simulink model "NXPFRDMK64F"  (R2022a)
settings: Solver=FixedStepAuto  StartTime=0.0  StopTime=10.0  FixedStep=1e-3  RelTol=1e-3  EnableMultiTasking=on
undefined symbols (not defined in the file): D0, D1, D10, D11, D12, D13, D2, D3, D4, D5, D6, D7, D8, D9, PTA0, PTA1, PTA2, PTB23, PTB9, PTC16, PTC17, PTC2, PTC3, PTC4, PTD0, PTD1, PTD2, PTD3
libraries: frdmk64flib x16
settings Model: ExtModeTrigDuration=5  Creator=patri  LastModifiedBy=areeb
settings OptimizationCC: EnhancedBackFolding=on  PassReuseOutputArgsAs=Individual arguments  ZeroExternalMemoryAtStartup=off  ZeroInternalMemoryAtStartup=off  MaxStackSize=64  OptimizeBlockOrder=speed  DifferentSizesBufferReuse=on  OptimizationCustomize=off  EfficientTunableParamExpr=on
settings DebuggingCC: ParameterTunabilityLossMsg=error
settings HardwareCC: ProdBitPerPointer=32  ProdBitPerSizeT=32  ProdBitPerPtrDiffT=32  ProdLargestAtomicInteger=Long  ProdLargestAtomicFloat=Double  ProdWordSize=32  ProdHWDeviceType=ARM Compatible->ARM Cortex
settings SFSimCC: MATLABDynamicMemAlloc=off
settings RTWCC: SystemTargetFile=ert.tlc  HardwareBoard=NXP FRDM-K64F  TLCOptions="-aInlineSetEventsForThisBaseRateFcn=TLC_FALSE -aSuppressMultiTaskScheduler=TLC_FALSE  -aRateBasedStepFcn=0"  TemplateMakefile=ert_default_tmf  Toolchain=GNU Tools for ARM Embedded Processors
settings CodeAppCC: ForceParamTrailComments=on  IgnoreCustomStorageClasses=off  OperatorAnnotations=on  SimulinkDataObjDesc=on  SFDataObjDesc=on  InsertBlockDesc=on
settings ERTTargetCC: ExtModeTransport=4  ExtModeMexFile=sendToCommService

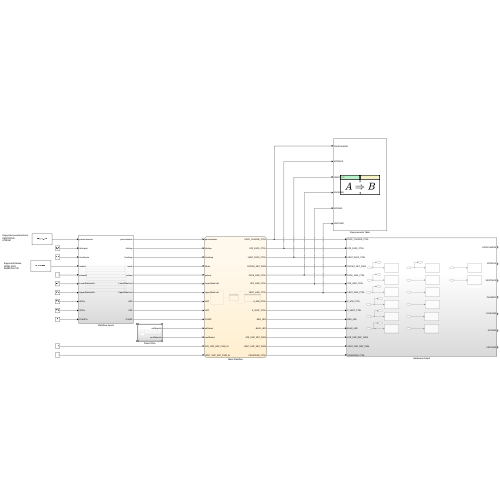
[thumbnail: Simulink's stored preview of the top-level diagram]
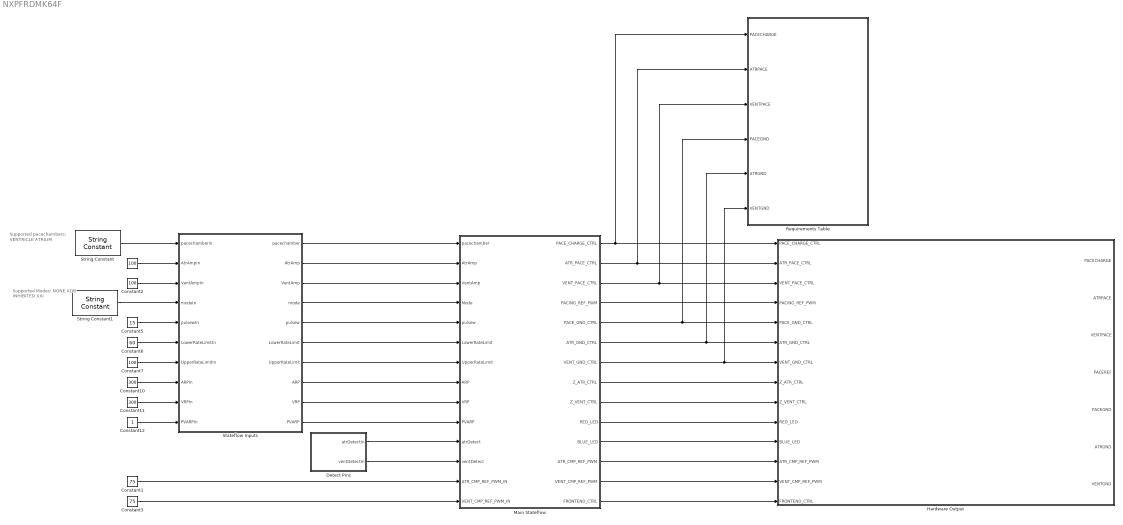
== system NXPFRDMK64F ==
  note: Supported pacechambers:
      | VENTRICLE
      | ATRIUM
  note: Supported Modes:
      | NONE XOO
      | INHIBITED XXI
  " " : Constant  Value=100
  Constant1 : Constant  Value=75
  Constant10 : Constant  Value=300
  Constant11 : Constant  Value=300
  Constant12 : Constant
  Constant2 : Constant  Value=100
  Constant3 : Constant  Value=75
  Constant5 : Constant  Value=15
  Constant6 : Constant  Value=60
  Constant7 : Constant  Value=100
  Detect Pins : Subsystem
  Hardware Output : Subsystem
  Main Stateflow : Stateflow chart  TreatAsAtomicUnit=on
  Requirements Table : Requirements Table  TreatAsAtomicUnit=on
  Stateflow Inputs : Subsystem
  String Constant : StringConstant  String="\"ATRIUM\""
  String Constant1 : StringConstant  String="\"INHIBITED\""
  wires:
  Main Stateflow/1(PACE_CHARGE_CTRL) -> Requirements Table/1(PACECHARGE), Hardware Output/1(PACE_CHARGE_CTRL)
  Main Stateflow/3(VENT_PACE_CTRL) -> Requirements Table/3(VENTPACE), Hardware Output/3(VENT_PACE_CTRL)
  Main Stateflow/4(PACING_REF_PWM) -> Hardware Output/4(PACING_REF_PWM)
  Main Stateflow/5(PACE_GND_CTRL) -> Requirements Table/4(PACEGND), Hardware Output/5(PACE_GND_CTRL)
  Main Stateflow/7(VENT_GND_CTRL) -> Requirements Table/6(VENTGND), Hardware Output/7(VENT_GND_CTRL)
  Main Stateflow/8(Z_ATR_CTRL) -> Hardware Output/8("Z_ATR_CTRL ")
  Main Stateflow/9(Z_VENT_CTRL) -> Hardware Output/9(Z_VENT_CTRL)
  Main Stateflow/11(BLUE_LED) -> Hardware Output/11(BLUE_LED)
  Main Stateflow/10(RED_LED) -> Hardware Output/10(RED_LED)
  Stateflow Inputs/1(pacechamber) -> Main Stateflow/1(pacechamber)
  Stateflow Inputs/2(AtrAmp) -> Main Stateflow/2(AtrAmp)
  Stateflow Inputs/3(VentAmp) -> Main Stateflow/3(VentAmp)
  Stateflow Inputs/4(mode) -> Main Stateflow/4(Mode)
  Stateflow Inputs/5(pulsew) -> Main Stateflow/5(pulsew)
  Stateflow Inputs/6(LowerRateLimit) -> Main Stateflow/6(LowerRateLimit)
  Stateflow Inputs/7(UpperRateLimit) -> Main Stateflow/7(UpperRateLimit)
  Stateflow Inputs/8(ARP) -> Main Stateflow/8(ARP)
  Stateflow Inputs/9(VRP) -> Main Stateflow/9(VRP)
  Stateflow Inputs/10(PVARP) -> Main Stateflow/10(PVARP)
  Detect Pins/1(atrDetectIn) -> Main Stateflow/11(atrDetect)
  Detect Pins/2(ventDetectIn) -> Main Stateflow/12(ventDetect)
  Constant12/1 -> Stateflow Inputs/10(PVARPIn)
  " "/1 -> Stateflow Inputs/2(AtrAmpIn)
  Constant2/1 -> Stateflow Inputs/3(VentAmpIn)
  String Constant1/1 -> Stateflow Inputs/4(modeIn)
  Constant5/1 -> Stateflow Inputs/5(pulsewIn)
  Constant6/1 -> Stateflow Inputs/6(LowerRateLimitIn)
  Constant7/1 -> Stateflow Inputs/7(UpperRateLimitIn)
  Constant10/1 -> Stateflow Inputs/8(ARPIn)
  Constant11/1 -> Stateflow Inputs/9(VRPIn)
  Constant1/1 -> Main Stateflow/13(ATR_CMP_REF_PWM_IN)
  Constant3/1 -> Main Stateflow/14(VENT_CMP_REF_PWM_IN)
  String Constant/1 -> Stateflow Inputs/1(pacechamberin)
  Main Stateflow/6(ATR_GND_CTRL) -> Requirements Table/5(ATRGND), Hardware Output/6(ATR_GND_CTRL)
  Main Stateflow/2(ATR_PACE_CTRL) -> Requirements Table/2(ATRPACE), Hardware Output/2(ATR_PACE_CTRL)
  Main Stateflow/12(ATR_CMP_REF_PWM) -> Hardware Output/12(ATR_CMP_REF_PWM)
  Main Stateflow/13(VENT_CMP_REF_PWM) -> Hardware Output/13(VENT_CMP_REF_PWM)
  Main Stateflow/14(FRONTEND_CTRL) -> Hardware Output/14(FRONTEND_CTRL)

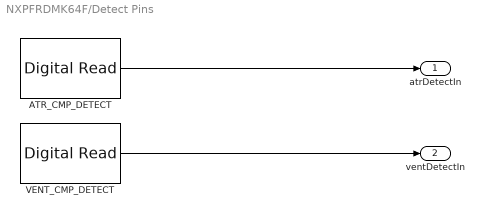
== system NXPFRDMK64F/Detect Pins ==
  ATR_CMP_DETECT : frdmk64flib/Digital Read  Whichpin=PTC16 (D0)  SampleTime=-1
  VENT_CMP_DETECT : frdmk64flib/Digital Read  Whichpin=PTC17 (D1)  SampleTime=-1
  atrDetectIn : Outport
  ventDetectIn : Outport  Port=2
  wires:
  VENT_CMP_DETECT/1 -> ventDetectIn/1
  ATR_CMP_DETECT/1 -> atrDetectIn/1

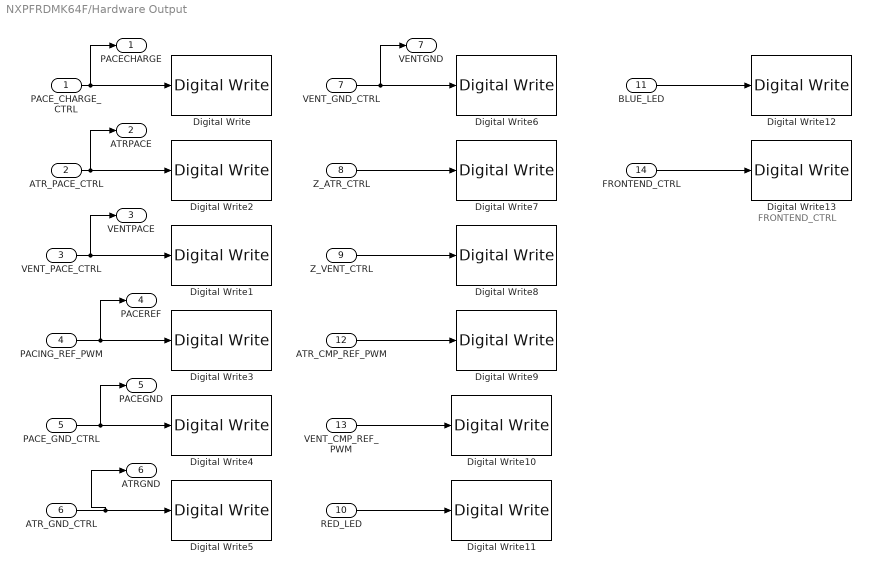
== system NXPFRDMK64F/Hardware Output ==
  note: FRONTEND_CTRL
  PACE_CHARGE_CTRL : Inport
  ATR_PACE_CTRL : Inport  Port=2
  VENT_PACE_CTRL : Inport  Port=3
  PACING_REF_PWM : Inport  Port=4
  PACE_GND_CTRL : Inport  Port=5
  ATR_GND_CTRL : Inport  Port=6
  VENT_GND_CTRL : Inport  Port=7
  "Z_ATR_CTRL " : Inport  Port=8
  Z_VENT_CTRL : Inport  Port=9
  RED_LED : Inport  Port=10
  BLUE_LED : Inport  Port=11
  ATR_CMP_REF_PWM : Inport  Port=12
  VENT_CMP_REF_PWM : Inport  Port=13
  FRONTEND_CTRL : Inport  Port=14
  Digital Write : frdmk64flib/Digital Write  Whichpin=PTB9 (D2)
  Digital Write1 : frdmk64flib/Digital Write  Whichpin=PTC4 (D9)
  Digital Write10 : frdmk64flib/Digital Write  Whichpin=PTA1 (D3)
  Digital Write11 : frdmk64flib/Digital Write  Whichpin=RED_LED
  Digital Write12 : frdmk64flib/Digital Write  Whichpin=BLUE_LED
  Digital Write13 : frdmk64flib/Digital Write  Whichpin=PTD1 (D13)
  Digital Write2 : frdmk64flib/Digital Write  Whichpin=PTA0 (D8)
  Digital Write3 : frdmk64flib/Digital Write  Whichpin=PTA2 (D5)
  Digital Write4 : frdmk64flib/Digital Write  Whichpin=PTD0 (D10)
  Digital Write5 : frdmk64flib/Digital Write  Whichpin=PTD2 (D11)
  Digital Write6 : frdmk64flib/Digital Write  Whichpin=PTD3 (D12)
  Digital Write7 : frdmk64flib/Digital Write  Whichpin=PTB23 (D4)
  Digital Write8 : frdmk64flib/Digital Write  Whichpin=PTC3 (D7)
  Digital Write9 : frdmk64flib/Digital Write  Whichpin=PTC2 (D6)
  PACECHARGE : Outport
  ATRPACE : Outport  Port=2
  VENTPACE : Outport  Port=3
  PACEREF : Outport  Port=4
  PACEGND : Outport  Port=5
  ATRGND : Outport  Port=6
  VENTGND : Outport  Port=7
  wires:
  "Z_ATR_CTRL "/1 -> Digital Write7/1
  ATR_CMP_REF_PWM/1 -> Digital Write9/1
  Z_VENT_CTRL/1 -> Digital Write8/1
  VENT_CMP_REF_PWM/1 -> Digital Write10/1
  BLUE_LED/1 -> Digital Write12/1
  PACE_CHARGE_CTRL/1 -> Digital Write/1, PACECHARGE/1
  RED_LED/1 -> Digital Write11/1
  ATR_PACE_CTRL/1 -> ATRPACE/1, Digital Write2/1
  VENT_PACE_CTRL/1 -> VENTPACE/1, Digital Write1/1
  PACING_REF_PWM/1 -> PACEREF/1, Digital Write3/1
  PACE_GND_CTRL/1 -> PACEGND/1, Digital Write4/1
  ATR_GND_CTRL/1 -> ATRGND/1, Digital Write5/1
  VENT_GND_CTRL/1 -> VENTGND/1, Digital Write6/1
  FRONTEND_CTRL/1 -> Digital Write13/1

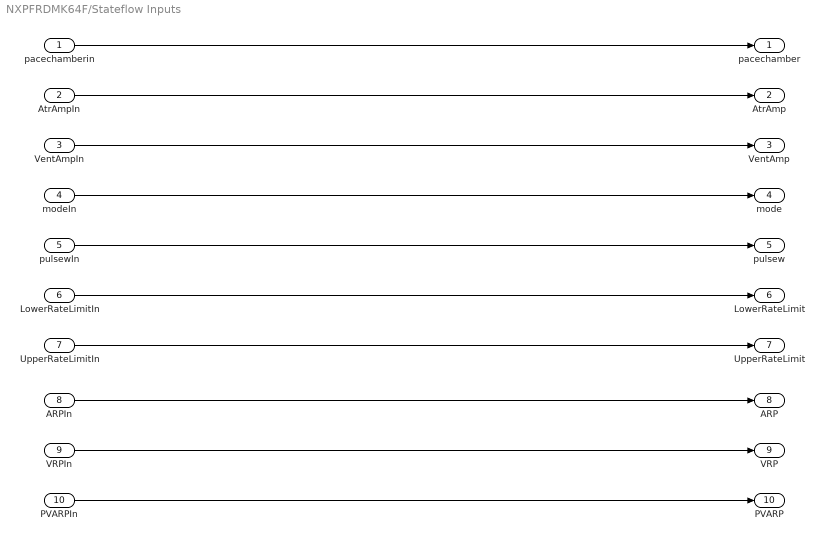
== system NXPFRDMK64F/Stateflow Inputs ==
  pacechamberin : Inport
  AtrAmpIn : Inport  Port=2
  VentAmpIn : Inport  Port=3
  modeIn : Inport  Port=4
  pulsewIn : Inport  Port=5
  LowerRateLimitIn : Inport  Port=6
  UpperRateLimitIn : Inport  Port=7
  ARPIn : Inport  Port=8
  VRPIn : Inport  Port=9
  PVARPIn : Inport  Port=10
  pacechamber : Outport
  AtrAmp : Outport  Port=2
  VentAmp : Outport  Port=3
  mode : Outport  Port=4
  pulsew : Outport  Port=5
  LowerRateLimit : Outport  Port=6
  UpperRateLimit : Outport  Port=7
  ARP : Outport  Port=8
  VRP : Outport  Port=9
  PVARP : Outport  Port=10
  wires:
  pacechamberin/1 -> pacechamber/1
  pulsewIn/1 -> pulsew/1
  modeIn/1 -> mode/1
  UpperRateLimitIn/1 -> UpperRateLimit/1
  LowerRateLimitIn/1 -> LowerRateLimit/1
  PVARPIn/1 -> PVARP/1
  AtrAmpIn/1 -> AtrAmp/1
  VentAmpIn/1 -> VentAmp/1
  ARPIn/1 -> ARP/1
  VRPIn/1 -> VRP/1

== stateflow chart NXPFRDMK64F/Requirements Table ==
  (default) -> (junction 1073742759)
  (junction 1073742759) -> (junction 1073742760) : {
      | % SF_REQ_REV_07
      | }
  (junction 1073742760) -> (junction 1073742762) : {
      | % HEADER_ASSIGNMENTS
      |
      | }
  (junction 1073742762) -> (junction 1073742764) : {
      | % START_A_4
      | }
  (junction 1073742764) -> (junction 1073742766) : {
      | }
  (junction 1073742766) -> (junction 1073742768)
  (junction 1073742768) -> (junction 1073742770) : {
      | }
  (junction 1073742770) -> (junction 1073742772) : {
      | % END_A_4
      | }
  (junction 1073742772) -> (junction 1073742774) : {
      | % START_R_1
      | }
  (junction 1073742774) -> (junction 1073742776) : {
      | }
  (junction 1073742776) -> (junction 1073742778)
  (junction 1073742778) -> (junction 1073742780) [order 1] : [duration((((PACECHARGE) == (0))) && (((ATRPACE) == (1))) && (((PACEGND) == (1))) && (((ATRGND) == (0))) && (((VENTGND) == (0)))) >= 1]
  (junction 1073742778) -> (junction 1073742786) [order 2]
  (junction 1073742780) -> (junction 1073742782) : {
      | true
      |
      | }
  (junction 1073742782) -> (junction 1073742784) : {
      | }
  (junction 1073742784) -> (junction 1073742786)
  (junction 1073742786) -> (junction 1073742788)
  (junction 1073742788) -> (junction 1073742790) : {
      | % END_R_1
      | }
  (junction 1073742790) -> (junction 1073742792) : {
      | % START_R_10
      | }
  (junction 1073742792) -> (junction 1073742794) : {
      | }
  (junction 1073742794) -> (junction 1073742796)
  (junction 1073742796) -> (junction 1073742798) [order 1] : [duration((((PACECHARGE) == (1))) && (((ATRPACE) == (0))) && (((VENTPACE) == (0))) && (((PACEGND) == (0))) && (((ATRGND) == (1))) && (((VENTGND) == (0)))) >= 1.015]
  (junction 1073742796) -> (junction 1073742804) [order 2]
  (junction 1073742798) -> (junction 1073742800) : {
      | true
      |
      | }
  (junction 1073742800) -> (junction 1073742802) : {
      | }
  (junction 1073742802) -> (junction 1073742804)
  (junction 1073742804) -> (junction 1073742806)
  (junction 1073742806) -> (junction 1073742808) : {
      | % END_R_10
      | }
  (junction 1073742808) -> (junction 1073742810) : {
      | % START_R_7
      | }
  (junction 1073742810) -> (junction 1073742812) : {
      | }
  (junction 1073742812) -> (junction 1073742814)
  (junction 1073742814) -> (junction 1073742816) [order 1] : [duration((((PACECHARGE) == (0))) && (((VENTPACE) == (1))) && (((PACEGND) == (1))) && (((ATRGND) == (0))) && (((VENTGND) == (0)))) >= 1]
  (junction 1073742814) -> (junction 1073742822) [order 2]
  (junction 1073742816) -> (junction 1073742818) : {
      | true
      |
      | }
  (junction 1073742818) -> (junction 1073742820) : {
      | }
  (junction 1073742820) -> (junction 1073742822)
  (junction 1073742822) -> (junction 1073742824)
  (junction 1073742824) -> (junction 1073742826) : {
      | % END_R_7
      | }
  (junction 1073742826) -> (junction 1073742828) : {
      | % START_R_13
      | }
  (junction 1073742828) -> (junction 1073742830) : {
      | }
  (junction 1073742830) -> (junction 1073742832)
  (junction 1073742832) -> (junction 1073742834) [order 1] : [duration((((PACECHARGE) == (1))) && (((ATRPACE) == (0))) && (((VENTPACE) == (0))) && (((PACEGND) == (0))) && (((ATRGND) == (0))) && (((VENTGND) == (1)))) >= 1.015]
  (junction 1073742832) -> (junction 1073742840) [order 2]
  (junction 1073742834) -> (junction 1073742836) : {
      | true
      |
      | }
  (junction 1073742836) -> (junction 1073742838) : {
      | }
  (junction 1073742838) -> (junction 1073742840)
  (junction 1073742840) -> (junction 1073742842)
  (junction 1073742842) -> (junction 1073742844) : {
      | % END_R_13
      | }
  data: PACECHARGE input; ATRPACE input; VENTPACE input; PACEGND input; ATRGND input; VENTGND input

== stateflow chart NXPFRDMK64F/Main Stateflow ==
  note: SensingStateflow
      | Holds the logic for sensing heart activity and responding to it. The letter code is considered before branching deeper based on the chamber sensed
  state Initialize
    FRONTEND_CTRL = true;
    ATR_CMP_REF_PWM = ATR_CMP_REF_PWM_IN;
    VENT_CMP_REF_PWM = VENT_CMP_REF_PWM_IN;
    %Reset LEDS
    RED_LED = false;
    BLUE_LED = false;
    Z_VENT_CTRL = false;
    Z_ATR_CTRL = false;
    % selecting correct initial pulse amplitude
    if pacechamber == "VENTRICLE"
    PulseAmp = VentAmp;
    PACING_REF_PWM = VENT_CMP_REF_PWM;
    else
    PulseAmp = AtrAmp;
    PACING_REF_PWM = ATR_CMP_REF_PWM;
    end
    %Set default values
    VENT_PACE_CTRL = false;
    ATR_PACE_CTRL = false;
    PACE_GND_CTRL = true;
    VENT_GND_CTRL = false;
    ATR_GND_CTRL = false;
    PACE_CHARGE_CTRL = true;
    DelayCarry = 0;
  note: PacingStateflow
      | Holds the logic for pacing each chamber.
  state Pace
    state AtriumPace
      ATR_PACE_CTRL = true;
      %LED to display state
      RED_LED = true;
    state ChargeC22_DischargeC21
      %Discharge C21
      %Ensure patient is never directly connect to PWM
      VENT_PACE_CTRL = false;
      ATR_PACE_CTRL = false;
      PACE_GND_CTRL = true;
      %Check for what chamber is to be paced
      if(Chamber == 0)
      ATR_GND_CTRL = true;
      VENT_GND_CTRL = false;
      else
      ATR_GND_CTRL = false;
      VENT_GND_CTRL = true;
      end
      %Charge C22
      if pacechamber == "VENTRICLE"
      PACING_REF_PWM = VENT_CMP_REF_PWM;
      else
      PACING_REF_PWM = ATR_CMP_REF_PWM;
      end
      PACE_CHARGE_CTRL = true;
      %LED "blinks" for each pace
      RED_LED = false;
      BLUE_LED = false;
      %Exit out to sense again
      send(endpace)
    note: 0 Atrium
        | 1 Ventricle
    state ClearSignal
      %Clear signal before pacing
      ATR_GND_CTRL = false;
      PACE_GND_CTRL = true;
      VENT_GND_CTRL = false;
      PACE_CHARGE_CTRL = false;
    state VentriclePace
      VENT_PACE_CTRL = true;
      %LED to display state
      BLUE_LED = true;
    AtriumPace -> ChargeC22_DischargeC21 : after(pulsew,msec)
        | {DelayCarry = pulsew}
    ClearSignal -> AtriumPace [order 1] : [Chamber == 0]
    (default) -> ClearSignal
    ClearSignal -> VentriclePace [order 2] : [Chamber ==1]
    VentriclePace -> ChargeC22_DischargeC21 : after(pulsew,msec)
        | {DelayCarry = pulsew}
  state Sense
    note: Default exists to constantly check if the mode is the same or is changed for the next cycle.
    note: Loops back for sensed case in inhibited
    note: Loops back for sensed case in inhibited
    note: Ventricle modes
    note: Atrium modes
    state Atrium
      note: Sets the active chamber, which directs where to pace
          | 0 = Atrium
          | 1 = Ventrical
      state None
        %Wait for a time then pace
        send(startpace)
      state Default
        Chamber = 0;
      state Pace
        send(startpace)
      state Inhibited
        %checks if the heart is already paced
        %Reset carry for the next cycle
        DelayCarry = 0;
        send(A_Loop)
      state Buffer
        %delay
      (default) -> Sense.Atrium.Default
      (junction 208) -> Sense.Atrium.None [order 1] : after(ARP,msec)
          | [Mode == "NONE"]
      Sense.Atrium.Default -> (junction 208)
      Sense.Atrium.Buffer -> Sense.Atrium.Pace [order 2] : after((60000/LowerRateLimit)-DelayCarry,msec)
      (junction 208) -> Sense.Atrium.Buffer [order 2] : after(ARP,msec)
          |  [Mode == "INHIBITED"]
          | {DelayCarry = DelayCarry+ARP}
      Sense.Atrium.Buffer -> Sense.Atrium.Inhibited [order 1] : [atrDetect]
    state Ventricle
      note: Sets the active chamber, which directs where to pace
          | 0 = Atrium
          | 1 = Ventrical
      state None
        %Wait for a time then pace
        send(startpace)
      state Default
        Chamber = 1;
      state Pace
        send(startpace)
      state Inhibited
        %checks if the heart is already paced
        %Reset carry for the next cycle
        DelayCarry = 0;
        send(V_Loop)
      state Buffer
        %delay
      (default) -> Sense.Ventricle.Default
      (junction 222) -> Sense.Ventricle.None [order 1] : after(VRP,msec)
          | [Mode == "NONE"]
      Sense.Ventricle.Default -> (junction 222)
      Sense.Ventricle.Buffer -> Sense.Ventricle.Pace [order 2] : after((60000/LowerRateLimit)-DelayCarry,msec)
      (junction 222) -> Sense.Ventricle.Buffer [order 2] : after(VRP,msec)
          |  [Mode == "INHIBITED"]
          | {DelayCarry = DelayCarry+VRP}
      Sense.Ventricle.Buffer -> Sense.Ventricle.Inhibited [order 1] : [ventDetect]
    state Default
    (default) -> Sense.Default
    Atrium -> Sense.Default : A_Loop
    Ventricle -> Sense.Default : V_Loop
    Sense.Default -> Atrium [order 2] : [pacechamber=="ATRIUM"]
    Sense.Default -> Ventricle [order 1] : [pacechamber=="VENTRICLE"]
  (default) -> Initialize
  Sense -> Pace : startpace
  Initialize -> Sense
  Pace -> Sense : endpace
  data: PACE_CHARGE_CTRL output; ATR_PACE_CTRL output; VENT_PACE_CTRL output; PACING_REF_PWM output; PACE_GND_CTRL output; ATR_GND_CTRL output; VENT_GND_CTRL output; Z_ATR_CTRL output; Z_VENT_CTRL output; pacechamber input; AtrAmp input; VentAmp input; Mode input; pulsew input; RED_LED output; BLUE_LED output; PulseAmp local; LowerRateLimit input; UpperRateLimit input; ARP input; VRP input; PVARP input; atrDetect input; ventDetect input; Chamber local; ATR_CMP_REF_PWM_IN input; VENT_CMP_REF_PWM_IN input; ATR_CMP_REF_PWM output; VENT_CMP_REF_PWM output; DelayCarry local; FRONTEND_CTRL output
  events: startpace local FUNCTION_CALL_EVENT; endpace local FUNCTION_CALL_EVENT; V_Loop local FUNCTION_CALL_EVENT; A_Loop local FUNCTION_CALL_EVENT
